simulink subsystem "PvtSubSys_HMI"  (R2020b)
settings: Solver=VariableStepAuto  StartTime=0.0  StopTime=10.0  RelTol=1e-3
undefined symbols (not defined in the file): P_HMI_LDW_LKAWarnTime, P_HMI_ObjectTypeFilter, P_HMI_WarnFormLDWReq
libraries: simulink x212, TrueDurationTime x6
(part 8 of 8)

== matlab function PvtSubSys_HMI/HMI2.12/IFC_Signal1/Subsystem50/MATLAB Function1 ==
  data: standstill input boolean; out output single; in input single; update input boolean; inrecorder input single; recorder output single
function [out,recorder] = fcn(standstill,in,update,inrecorder)
recorder=inrecorder;
out=single(0);
if update%当车辆由运动到静止时记录recorder，并在车辆运动时将recorder清零
    recorder=in;
end
if standstill==0%车辆运动时采用实际值，车辆静止时采用recorder值
    out=in;
elseif standstill==1
    if update
        out=in;
    else
        out=inrecorder;
    end
end

== matlab function PvtSubSys_HMI/HMI2.12/IFC_Signal1/Subsystem51/MATLAB Function1 ==
  data: standstill input boolean; out output single; in input single; update input boolean; inrecorder input single; recorder output single
function [out,recorder] = fcn(standstill,in,update,inrecorder)
recorder=inrecorder;
out=single(0);
if update%当车辆由运动到静止时记录recorder，并在车辆运动时将recorder清零
    recorder=in;
end
if standstill==0%车辆运动时采用实际值，车辆静止时采用recorder值
    out=in;
elseif standstill==1
    if update
        out=in;
    else
        out=inrecorder;
    end
end

== matlab function PvtSubSys_HMI/HMI2.12/IFC_Signal1/Subsystem52/MATLAB Function1 ==
  data: standstill input boolean; out output single; in input single; update input boolean; inrecorder input single; recorder output single
function [out,recorder] = fcn(standstill,in,update,inrecorder)
recorder=inrecorder;
out=single(0);
if update%当车辆由运动到静止时记录recorder，并在车辆运动时将recorder清零
    recorder=in;
end
if standstill==0%车辆运动时采用实际值，车辆静止时采用recorder值
    out=in;
elseif standstill==1
    if update
        out=in;
    else
        out=inrecorder;
    end
end

== matlab function PvtSubSys_HMI/HMI2.12/IFC_Signal1/MATLAB Function13 ==
  data: fType input; Type output
function Type = fcn(fType)

Type=fType;
if fType==14||fType==20
    Type=uint8(2);
end

== matlab function PvtSubSys_HMI/HMI2.12/IFC_Signal1/Subsystem54/MATLAB Function1 ==
  data: standstill input boolean; out output single; in input single; update input boolean; inrecorder input single; recorder output single
function [out,recorder] = fcn(standstill,in,update,inrecorder)
recorder=inrecorder;
out=single(0);
if update%当车辆由运动到静止时记录recorder，并在车辆运动时将recorder清零
    recorder=in;
end
if standstill==0%车辆运动时采用实际值，车辆静止时采用recorder值
    out=in;
elseif standstill==1
    if update
        out=in;
    else
        out=inrecorder;
    end
end

== matlab function PvtSubSys_HMI/HMI2.12/HWA//ACC//TJA_Signal1/MATLAB Function3 ==
  data: HWASts input; LaneChange output
function LaneChange = fcn(HWASts)
LaneChange=uint8(0);
if HWASts==5
    LaneChange=uint8(1);
elseif HWASts==6
    LaneChange=uint8(2);
end

== matlab function PvtSubSys_HMI/HMI2.12/IFC_Signal1/Subsystem55/MATLAB Function1 ==
  data: standstill input boolean; out output single; in input single; update input boolean; inrecorder input single; recorder output single
function [out,recorder] = fcn(standstill,in,update,inrecorder)
recorder=inrecorder;
out=single(0);
if update%当车辆由运动到静止时记录recorder，并在车辆运动时将recorder清零
    recorder=in;
end
if standstill==0%车辆运动时采用实际值，车辆静止时采用recorder值
    out=in;
elseif standstill==1
    if update
        out=in;
    else
        out=inrecorder;
    end
end

== matlab function PvtSubSys_HMI/HMI2.12/IFC_Signal1/Subsystem56/MATLAB Function1 ==
  data: standstill input boolean; out output uint8; in input uint8; update input boolean; inrecorder input uint8; recorder output uint8
function [out,recorder] = fcn(standstill,in,update,inrecorder)
recorder=inrecorder;
out=uint8(0);
if update%当车辆由运动到静止时记录recorder，并在车辆运动时将recorder清零
    recorder=in;
end
if standstill==0%车辆运动时采用实际值，车辆静止时采用recorder值
    out=in;
elseif standstill==1
    if update
        out=in;
    else
        out=inrecorder;
    end
end

== matlab function PvtSubSys_HMI/HMI2.12/IFC_Signal1/Subsystem57/MATLAB Function1 ==
  data: standstill input boolean; out output uint8; in input uint8; update input boolean; inrecorder input uint8; recorder output uint8
function [out,recorder] = fcn(standstill,in,update,inrecorder)
recorder=inrecorder;
out=uint8(0);
if update%当车辆由运动到静止时记录recorder，并在车辆运动时将recorder清零
    recorder=in;
end
if standstill==0%车辆运动时采用实际值，车辆静止时采用recorder值
    out=in;
elseif standstill==1
    if update
        out=in;
    else
        out=inrecorder;
    end
end

== matlab function PvtSubSys_HMI/HMI2.12/IFC_Signal1/Subsystem58/MATLAB Function1 ==
  data: standstill input boolean; out output uint8; in input uint8; update input boolean; inrecorder input uint8; recorder output uint8
function [out,recorder] = fcn(standstill,in,update,inrecorder)
recorder=inrecorder;
out=uint8(0);
if update%当车辆由运动到静止时记录recorder，并在车辆运动时将recorder清零
    recorder=in;
end
if standstill==0%车辆运动时采用实际值，车辆静止时采用recorder值
    out=in;
elseif standstill==1
    if update
        out=in;
    else
        out=inrecorder;
    end
end

== matlab function PvtSubSys_HMI/HMI2.12/IFC_Signal1/Subsystem59/MATLAB Function1 ==
  data: standstill input boolean; out output single; in input single; update input boolean; inrecorder input single; recorder output single
function [out,recorder] = fcn(standstill,in,update,inrecorder)
recorder=inrecorder;
out=single(0);
if update%当车辆由运动到静止时记录recorder，并在车辆运动时将recorder清零
    recorder=in;
end
if standstill==0%车辆运动时采用实际值，车辆静止时采用recorder值
    out=in;
elseif standstill==1
    if update
        out=in;
    else
        out=inrecorder;
    end
end

== matlab function PvtSubSys_HMI/HMI2.12/HWA//ACC//TJA_Signal1/MATLAB Function4 ==
  data: AngRaw input single; Angle output single
function Angle = AngCalc(AngRaw)
if AngRaw>1.57
    Angle = AngRaw - single(3.14);
elseif AngRaw<-1.57
    Angle = AngRaw + single(3.14);
else
    Angle = AngRaw;
end
